simulink model "problem2suspension"  (R2020b)
settings: Solver=VariableStepAuto  StartTime=0.0  StopTime=10.0  RelTol=1e-3
settings Model: Creator=Shivashis  LastModifiedBy=Shivashis

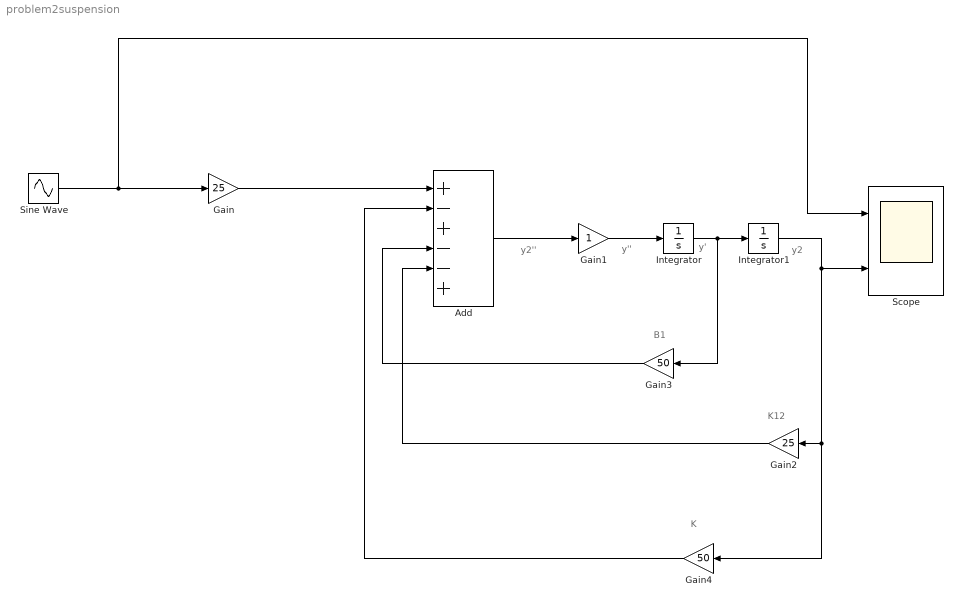
== system problem2suspension ==
  note: y2
  note: y'
  note: y''
  note: y2''
  note: K12
  note: B1
  note: K
  Add : Sum  Inputs=+-+--+
  Gain : Gain  Gain=25
  Gain1 : Gain
  Gain2 : Gain  Gain=25
  Gain3 : Gain  Gain=50
  Gain4 : Gain  Gain=50
  Integrator : Integrator
  Integrator1 : Integrator
  Scope : Scope  NumInputPorts=2
  Sine Wave : Sin  SampleTime=0
  wires:
  Gain/1 -> Add/1
  Add/1 -> Gain1/1
  Gain1/1 -> Integrator/1
  Integrator/1 -> Gain3/1, Integrator1/1
  Integrator1/1 -> Gain4/1, Gain2/1, Scope/2
  Gain4/1 -> Add/2
  Gain3/1 -> Add/4
  Gain2/1 -> Add/5
  Sine Wave/1 -> Scope/1, Gain/1
